simulink model "subsampling"  (R2025b)
settings: Solver=FixedStepAuto  StartTime=0.0  StopTime=9.999  RelTol=1e-3
model workspace (MAT data in the model file):
  Ts = 0.001
libraries: subsystems x4, simulink x3
settings Model: Creator=karadeli  LastModifiedBy=karadeli

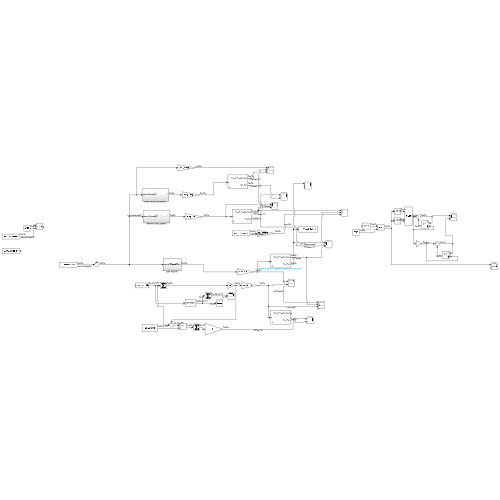
[thumbnail: Simulink's stored preview of the top-level diagram]
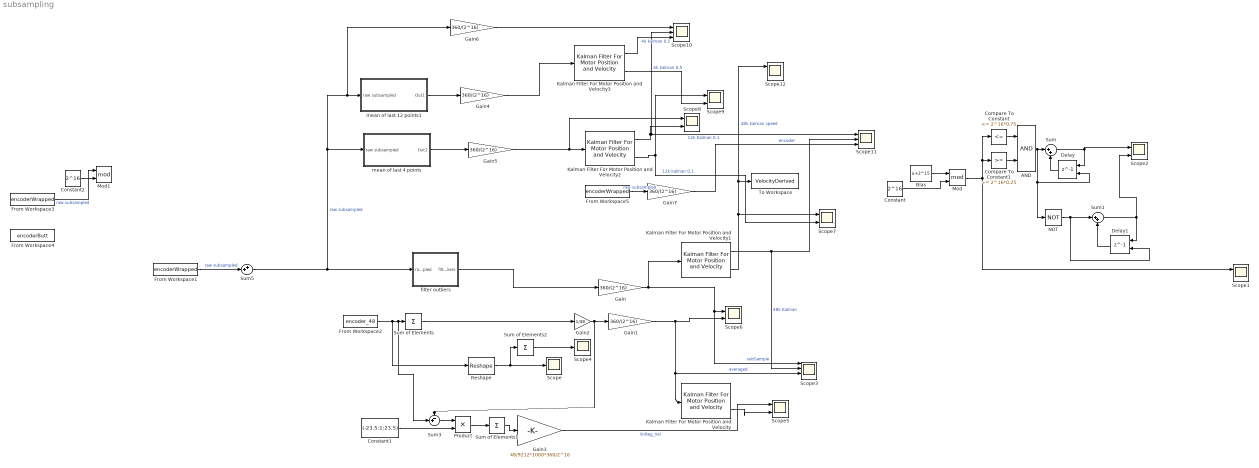
== system subsampling ==
  AND : Logic  AllPortsSameDT=off  OutDataTypeStr=boolean
  Bias : Bias  Bias=2^15  SaturateOnIntegerOverflow=off
  Compare To Constant : simulink/Logic and Bit Operations/Compare To Constant  relop=<=  const=2^16*0.75  OutDataTypeStr=boolean
  Compare To Constant1 : simulink/Logic and Bit Operations/Compare To Constant  relop=>=  const=2^16*0.25  OutDataTypeStr=boolean
  Constant : Constant  Value=2^16
  Constant1 : Constant  Value=(-23.5:1:23.5)
  Constant2 : Constant  Value=2^16
  Delay : Delay  DelayLength=1  ExternalReset=Falling
      settings: InputPortMap=u0,r5
  Delay1 : Delay  DelayLength=1  ExternalReset=Falling
      settings: InputPortMap=u0,r5
  From Workspace1 : FromWorkspace  VariableName=encoderWrapped  OutDataTypeStr=double  SampleTime=1e-3/48  Interpolate=off  OutputAfterFinalValue=Holding final value
  From Workspace2 : FromWorkspace  VariableName=encoder_48  SampleTime=1e-3  Interpolate=off  OutputAfterFinalValue=Holding final value
  From Workspace3 : FromWorkspace  VariableName=encoderWrapped  OutDataTypeStr=double  SampleTime=1e-3/48  Interpolate=off  OutputAfterFinalValue=Holding final value
  From Workspace4 : FromWorkspace  VariableName=encoderButt  OutDataTypeStr=double  SampleTime=1e-3  Interpolate=off  OutputAfterFinalValue=Holding final value
  From Workspace5 : FromWorkspace  VariableName=encoderWrapped  OutDataTypeStr=double  SampleTime=1e-3/48  Interpolate=off  OutputAfterFinalValue=Holding final value
  Gain{,1,4..7} (6 alike) : Gain  Gain=360/(2^16)
  Gain2 : Gain  Gain=1/48
  Gain3 : Gain  Gain=48/9212*1000*360/2^16
  Kalman Filter For Motor Position and Velocity : subsystems/Kalman Filter For Motor Position and Velocity  Ts=1e-3  lambda_RQ=1
  Kalman Filter For Motor Position and Velocity1 : subsystems/Kalman Filter For Motor Position and Velocity  Ts=1e-3/48  lambda_RQ=0.01
  Kalman Filter For Motor Position and Velocity2 : subsystems/Kalman Filter For Motor Position and Velocity  Ts=1e-3/12  lambda_RQ=0.1
  Kalman Filter For Motor Position and Velocity3 : subsystems/Kalman Filter For Motor Position and Velocity  Ts=1e-3/4  lambda_RQ=0.5
  Mod : Math  Operator=mod
  Mod1 : Math  Operator=mod
  NOT : Logic  Operator=NOT  IconShape=distinctive  AllPortsSameDT=off  OutDataTypeStr=boolean
  Product : Product
  Reshape : Reshape  OutputDimensionality=Customize  OutputDimensions=[4,12]
  Scope : Scope
  Scope{1..2,5..9} (7 alike) : Scope  NumInputPorts=2
      Scope1 settings: ActiveDisplayYMinimum=-3408.1618255270005  ActiveDisplayYMaximum=69223.077166894145
      Scope2 settings: ActiveDisplayYMinimum=-51.551724137930933  ActiveDisplayYMaximum=117.53793103448265  DataLoggingVariableName=ScopeData2
      Scope5 settings: ActiveDisplayYMinimum=-37903.757690281527  ActiveDisplayYMaximum=38085.635569249935  DataLoggingVariableName=ScopeData5
      Scope6 settings: ActiveDisplayYMinimum=-2765.3549194335938  ActiveDisplayYMaximum=-2718.3609008789062  DataLoggingVariableName=ScopeData6
      Scope7 settings: ActiveDisplayYMinimum=35846.916775025675  ActiveDisplayYMaximum=52037.05237399305  DataLoggingVariableName=ScopeData7
      Scope8 settings: ActiveDisplayYMinimum=17339.152462075763  ActiveDisplayYMaximum=17768.734796192097  DataLoggingVariableName=ScopeData8
      Scope9 settings: ActiveDisplayYMinimum=19765.389066033807  ActiveDisplayYMaximum=36488.892004121153  DataLoggingVariableName=ScopeData9
  Scope10 : Scope  NumInputPorts=3
      settings: ActiveDisplayYMinimum=-1825.5733501968643  ActiveDisplayYMaximum=-1702.5526945610532  DataLoggingVariableName=ScopeData10
  Scope11 : Scope  NumInputPorts=3
      settings: ActiveDisplayYMinimum=3878.3003880216247  ActiveDisplayYMaximum=4404.1000578739377  DataLoggingVariableName=ScopeData11
  Scope12 : Scope  NumInputPorts=3
      settings: ActiveDisplayYMinimum=38173.065657463412  ActiveDisplayYMaximum=51298.947723919955  DataLoggingVariableName=ScopeData12
  Scope3 : Scope  NumInputPorts=4
      settings: ActiveDisplayYMinimum=17464.694613932097  ActiveDisplayYMaximum=17576.915838252935  DataLoggingVariableName=ScopeData3
  Scope4 : Scope
      settings: ActiveDisplayYMinimum=-1  ActiveDisplayYMaximum=1  DataLoggingVariableName=ScopeData4
  Sum : Sum  Inputs=|++
  Sum of Elements : Sum  Inputs=+
  Sum of Elements1 : Sum  Inputs=+
  Sum of Elements2 : Sum  Inputs=+  CollapseMode=Specified dimension
  Sum1 : Sum  Inputs=|++
  Sum3 : Sum  Inputs=-+|
  Sum5 : Sum  Inputs=++|
  To Workspace : ToWorkspace  VariableName=VelocityDerived  SaveFormat=Timeseries  SampleTime=1e-3
  filter outliers : Subsystem
  mean of last 12 points1 : Subsystem
  mean of last 4 points : Subsystem
  wires:
  Bias/1 -> Mod/1
  Constant/1 -> Mod/2
  Mod/1 -> Compare To Constant/1, Compare To Constant1/1, Scope1/1
  Compare To Constant/1 -> AND/1
  Compare To Constant1/1 -> AND/2
  AND/1 -> NOT/1, Delay/2, Sum/1
  Delay/1 -> Sum/2
  Sum/1 -> Delay/1, Scope2/1
  NOT/1 -> Delay1/2, Sum1/1
  Sum1/1 -> Delay1/1, Scope2/2
  Delay1/1 -> Sum1/2
  Sum5/1 -> Gain6/1, mean of last 12 points1/1(raw subsampled), mean of last 4 points/1(raw subsampled), filter outliers/1(raw subsampled)  "raw subsampled"
  Gain/1 -> Scope3/1, Scope6/1, Kalman Filter For Motor Position and Velocity1/1  "subSample"
  Sum of Elements/1 -> Gain2/1
  Gain2/1 -> Sum3/1, Gain1/1
  Gain1/1 -> Scope3/3, Kalman Filter For Motor Position and Velocity/1, Scope6/2  "averaged"
  Kalman Filter For Motor Position and Velocity1/1 -> Scope3/2, Scope11/2  "48k Kalman"
  Kalman Filter For Motor Position and Velocity/2 -> Scope5/2
  From Workspace2/1 -> Reshape/1, Sum3/2, Sum of Elements/1
  Constant1/1 -> Product/2
  Sum3/1 -> Product/1
  Product/1 -> Sum of Elements1/1
  Gain3/1 -> Scope5/1  "linReg_Vel"
  Sum of Elements1/1 -> Gain3/1
  Kalman Filter For Motor Position and Velocity1/2 -> Scope12/1, To Workspace/1, Scope7/1  "48k kalman speed"
  Reshape/1 -> Sum of Elements2/1, Scope/1
  Sum of Elements2/1 -> Scope4/1
  Gain5/1 -> Scope8/1, Kalman Filter For Motor Position and Velocity2/1
  Kalman Filter For Motor Position and Velocity2/1 -> Scope10/2, Scope11/1, Scope8/2  "12k Kalman 0.1"
  Kalman Filter For Motor Position and Velocity2/2 -> Scope7/2, Scope9/1  "12k kalman 0.1"
  From Workspace3/1 -> Mod1/1  "raw subsampled"
  Constant2/1 -> Mod1/2
  From Workspace1/1 -> Sum5/2  "raw subsampled"
  From Workspace5/1 -> Gain7/1  "raw subsampled"
  Gain7/1 -> Scope11/3  "encoder"
  filter outliers/1(filter outliers) -> Gain/1
  mean of last 4 points/1(Out1) -> Gain5/1
  Kalman Filter For Motor Position and Velocity3/2 -> Scope9/2  "4k kalman 0.5"
  mean of last 12 points1/1(Out1) -> Gain4/1
  Gain4/1 -> Kalman Filter For Motor Position and Velocity3/1
  Kalman Filter For Motor Position and Velocity3/1 -> Scope10/3  "4k kalman 0.5"
  Gain6/1 -> Scope10/1

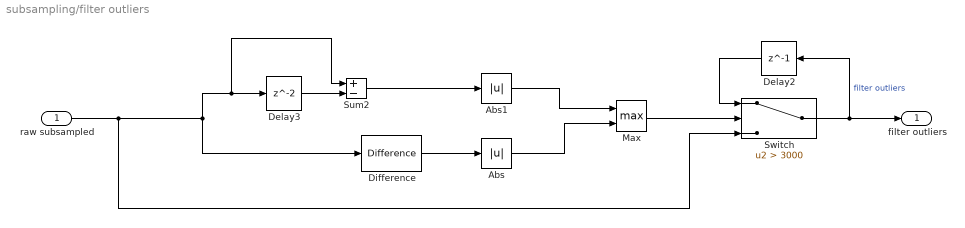
== system subsampling/filter outliers ==
  raw subsampled : Inport
  Abs : Abs  SaturateOnIntegerOverflow=off
  Abs1 : Abs  SaturateOnIntegerOverflow=off
  Delay2 : Delay  DelayLength=1  SampleTime=1e-3/48
  Delay3 : Delay
  Difference : simulink/Discrete/Difference  ICPrevInput=0.0  OutMin=[]  OutMax=[]  OutDataType=fixdt(1, 16)  OutScaling=2^-10  DoSatur=off
  Max : MinMax  Function=max  Inputs=2
  Sum2 : Sum  Inputs=+-
  Switch : Switch  Criteria=u2 > Threshold  Threshold=3000  SaturateOnIntegerOverflow=off  InputSameDT=off
  filter outliers : Outport
  wires:
  Difference/1 -> Abs/1
  Abs1/1 -> Max/1
  Abs/1 -> Max/2
  Max/1 -> Switch/2
  raw subsampled/1 -> Difference/1, Sum2/1, Delay3/1, Switch/3
  Delay3/1 -> Sum2/2
  Switch/1 -> filter outliers/1, Delay2/1  "filter outliers"
  Sum2/1 -> Abs1/1
  Delay2/1 -> Switch/1

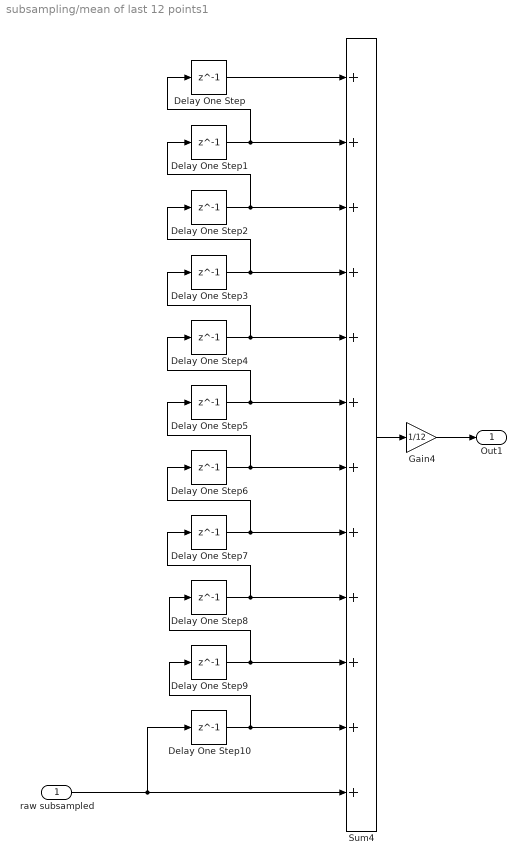
== system subsampling/mean of last 12 points1 ==
  raw subsampled : Inport
  Delay One Step{,1..10} (11 alike) : Delay  DelayLength=1
  Gain4 : Gain  Gain=1/12
  Sum4 : Sum  Inputs=12
  Out1 : Outport
  wires:
  Sum4/1 -> Gain4/1
  Gain4/1 -> Out1/1
  raw subsampled/1 -> Sum4/12, Delay One Step10/1
  Delay One Step8/1 -> Sum4/9, Delay One Step7/1
  Delay One Step7/1 -> Sum4/8, Delay One Step6/1
  Delay One Step6/1 -> Sum4/7, Delay One Step5/1
  Delay One Step5/1 -> Sum4/6, Delay One Step4/1
  Delay One Step4/1 -> Sum4/5, Delay One Step3/1
  Delay One Step3/1 -> Sum4/4, Delay One Step2/1
  Delay One Step2/1 -> Sum4/3, Delay One Step1/1
  Delay One Step1/1 -> Sum4/2, Delay One Step/1
  Delay One Step/1 -> Sum4/1
  Delay One Step9/1 -> Sum4/10, Delay One Step8/1
  Delay One Step10/1 -> Sum4/11, Delay One Step9/1

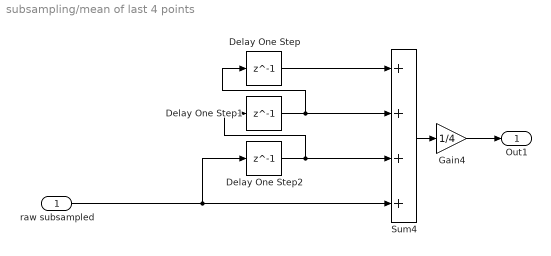
== system subsampling/mean of last 4 points ==
  raw subsampled : Inport
  Delay One Step : Delay  DelayLength=1
  Delay One Step1 : Delay  DelayLength=1
  Delay One Step2 : Delay  DelayLength=1
  Gain4 : Gain  Gain=1/4
  Sum4 : Sum  Inputs=++++
  Out1 : Outport
  wires:
  Gain4/1 -> Out1/1
  Delay One Step/1 -> Sum4/1
  Sum4/1 -> Gain4/1
  Delay One Step1/1 -> Delay One Step/1, Sum4/2
  raw subsampled/1 -> Delay One Step2/1, Sum4/4
  Delay One Step2/1 -> Delay One Step1/1, Sum4/3
